simulink model "radia_peec_coil_ac_plant"  (R2026a)
settings: Solver=FixedStepDiscrete  StopTime=0  FixedStep=1
PreLoadFcn:
  | R_coil_Ohm=0.02; X_coil_Ohm=0.05;
undefined symbols (not defined in the file or in its folder): C_F, f_eval_Hz, L_eff_H
settings Model: Creator=Administrator  LastModifiedBy=Administrator

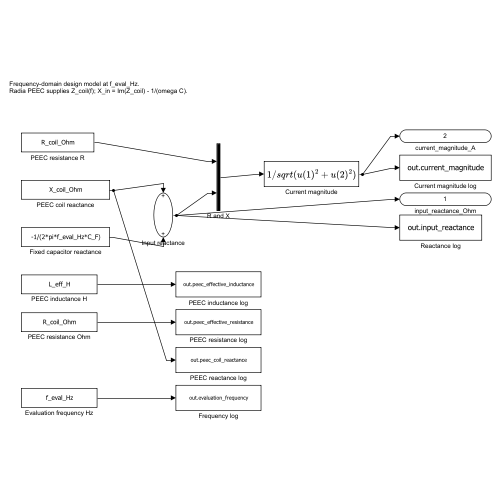
[thumbnail: Simulink's stored preview of the top-level diagram]
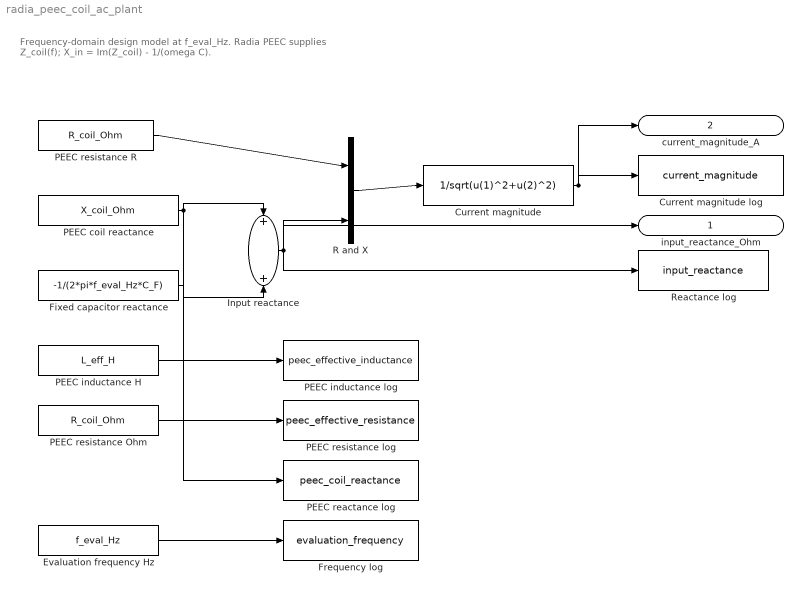
== system radia_peec_coil_ac_plant ==
  note: Frequency-domain design model at f_eval_Hz.
      | Radia PEEC supplies Z_coil(f); X_in = Im(Z_coil) - 1/(omega C).
  Current magnitude : Fcn  Expr=1/sqrt(u(1)^2+u(2)^2)
  Current magnitude log : ToWorkspace  VariableName=current_magnitude  SaveFormat=Timeseries  SampleTime=-1
  Evaluation frequency Hz : Constant  Value=f_eval_Hz
  Fixed capacitor reactance : Constant  Value=-1/(2*pi*f_eval_Hz*C_F)
  Frequency log : ToWorkspace  VariableName=evaluation_frequency  SaveFormat=Timeseries  SampleTime=-1
  Input reactance : Sum
  PEEC coil reactance : Constant  Value=X_coil_Ohm
  PEEC inductance H : Constant  Value=L_eff_H
  PEEC inductance log : ToWorkspace  VariableName=peec_effective_inductance  SaveFormat=Timeseries  SampleTime=-1
  PEEC reactance log : ToWorkspace  VariableName=peec_coil_reactance  SaveFormat=Timeseries  SampleTime=-1
  PEEC resistance Ohm : Constant  Value=R_coil_Ohm
  PEEC resistance R : Constant  Value=R_coil_Ohm
  PEEC resistance log : ToWorkspace  VariableName=peec_effective_resistance  SaveFormat=Timeseries  SampleTime=-1
  R and X : Mux  Inputs=2
  Reactance log : ToWorkspace  VariableName=input_reactance  SaveFormat=Timeseries  SampleTime=-1
  input_reactance_Ohm : Outport
  current_magnitude_A : Outport  Port=2
  wires:
  PEEC coil reactance/1 -> Input reactance/1, PEEC reactance log/1
  Fixed capacitor reactance/1 -> Input reactance/2
  PEEC resistance R/1 -> R and X/1
  Input reactance/1 -> R and X/2, Reactance log/1, input_reactance_Ohm/1
  R and X/1 -> Current magnitude/1
  Current magnitude/1 -> Current magnitude log/1, current_magnitude_A/1
  PEEC inductance H/1 -> PEEC inductance log/1
  PEEC resistance Ohm/1 -> PEEC resistance log/1
  Evaluation frequency Hz/1 -> Frequency log/1
